simulink model "Match"  (R2014b)
settings: Solver=ode45  StartTime=0.0  StopTime=10.0  RelTol=1e-3
libraries: simulink x1
settings Model: Creator=Jackie  LastModifiedBy=Jackie

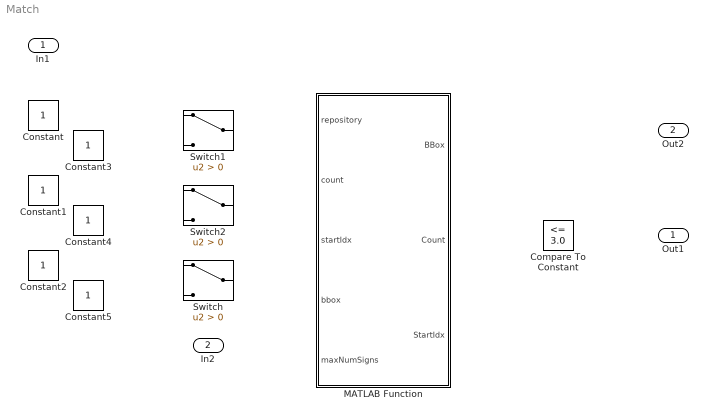
== system Match ==
  In1 : Inport
  In2 : Inport  Port=2
  Compare To Constant : simulink/Logic and Bit Operations/Compare To Constant  relop=<=  const=3.0  OutDataTypeStr=boolean
  Constant{,1..5} (6 alike) : Constant
  MATLAB Function : MATLAB Function  TreatAsAtomicUnit=on
  Switch : Switch  Criteria=u2 > Threshold
  Switch1 : Switch  Criteria=u2 > Threshold
  Switch2 : Switch  Criteria=u2 > Threshold
  Out1 : Outport
  Out2 : Outport  Port=2

== matlab function Match/MATLAB Function ==
  data: repository input; BBox output; count input; startIdx input; bbox input; maxNumSigns input; Count output; StartIdx output
function [BBox, Count, StartIdx] = Match(repository, count, startIdx, bbox, maxNumSigns)
% This function matches the targets found in the current video frame with
% those found in the previous frame. Targets in two video frames match
% when their bounding boxes overlap.
%
% Input:
%    repository: 
%       Bounding boxes of the targets found in the previous
%       frame. Each column has the format of [r, c, h, w] and corresponds 
%       to a target.
%    count: 
%       Number of video frames the target in the previous frame has 
%       been found.
%    startIdx: 
%       Index for the first new target in the current frame.
%    bbox: 
%       Bounding boxes of the targets found in the current frame.
%
% Output:
%    BBox: 
%       Bounding boxes of the targets found in the current frame. They
%       are ordered to have the same indices as their matching ones in the
%       previous frame.
%    Count: 
%       Number of video frames the target in the current frame has 
%       been found.
%    StartIdx: 
%       Index for the first new target in the next frame.

numBBox = single(size(bbox, 1));
BBox = single(zeros(maxNumSigns, 4));
Count = single(zeros(maxNumSigns,1));
impossible = single(10000); % A very large value
thr = single(2);
disMatrix = single(ones(maxNumSigns, numBBox)) * impossible;

% Calculate the distances between the repository and the current targets
for idx = single(1): maxNumSigns
    if repository(idx,3)>0 && repository(idx,4)>0
        for jdx = 1: numBBox
            if bbox(jdx,3)>0 && bbox(jdx,4)>0
                disMatrix(idx, jdx)...
                    = single(abs(2*(repository(idx,1)-bbox(jdx,1))...
                        +repository(idx,3)-bbox(jdx,3))...
                        / (repository(idx,3)+bbox(jdx,3))...
                        + abs(2*(repository(idx,2)-bbox(jdx,2))...
                        +repository(idx,4)-bbox(jdx,4))...
                        / (repository(idx,4)+bbox(jdx,4)));
            end
        end
    end
end

% Find the most similar pair of corners
for n = single(1): numBBox
    minVal = impossible;
    minIdx = single(0);
    minJdx = single(0);
    for idx = 1: single(maxNumSigns)
        for jdx = 1: numBBox
            if disMatrix(idx, jdx) < minVal
                minVal = disMatrix(idx, jdx);
                minIdx = idx;
                minJdx = jdx;
            end
        end
    end
    
    % Move the targets in the current frame so they have the same ordering
    % as their matching ones in the previous frame.
    if minVal < thr
        disMatrix(minIdx, :) = impossible;
        disMatrix(:, minJdx) = impossible;
        BBox(minIdx,:) = bbox(minJdx,:);
        Count(minIdx) = count(minIdx) + 1;
        bbox(minJdx,:) = single(zeros(4, 1));
    else
        break;
    end
end

% Copy the new targets
StartIdx = startIdx;
for jdx = single(1): numBBox
    if bbox(jdx,3)>0
        while BBox(StartIdx,3)
            if StartIdx<maxNumSigns
                StartIdx = StartIdx + single(1);
            else
                StartIdx = single(1);
            end
        end
        BBox(StartIdx, :) = bbox(jdx,:);
        Count(StartIdx) = single(1);
        if StartIdx<maxNumSigns
            StartIdx = StartIdx + single(1);
        else
            StartIdx = single(1);
        end
    end
end
